simulink model "Control_Schematic_12"  (Simulink 8.3)
settings: Solver=ode4  StartTime=0.0  StopTime=35  FixedStep=Ts  RelTol=1e-3
values from neighbouring files (symbols this model uses):
  Aob1 = Am1 - Lob1'*Cm1    [StartUp_12.m]    (also in StartUp_12a.m)
  Aob2 = Am2 - Lob2'*Cm2    [StartUp_12.m]    (also in StartUp_12a.m)
  b = 156    [StartUp_10_Validation.m]    (also in StartUp_12.m; StartUp_12a.m; StartUp_2.m; StartUp_5.m)
  Bob1 = [Bm1 Lob1']    [StartUp_12.m]    (also in StartUp_12a.m)
  Bob2 = [Bm2 Lob2']    [StartUp_12.m]    (also in StartUp_12a.m)
  Cob1 = [1 0 0;0 1 0]    [StartUp_12.m]    (also in StartUp_12a.m)
  Cob2 = [1 0 0;0 1 0]    [StartUp_12.m]    (also in StartUp_12a.m)
  Dob1 = zeros(2,2)    [StartUp_12.m]    (also in StartUp_12a.m)
  Dob2 = zeros(2,2)    [StartUp_12.m]    (also in StartUp_12a.m)
  r = 50    [StartUp_10_Validation.m]    (also in StartUp_12.m; StartUp_12a.m; StartUp_2.m = 820; StartUp_5.m = 0.01)
  Ts = 1/100    (= 0.01)    [StartUp_10_Validation.m]    (also in StartUp_12.m; StartUp_12a.m; StartUp_2.m = 0.001; StartUp_5.m = 0.001)
undefined symbols (not defined in the file or in its folder): Beta_Correction
undefined symbols (not defined in the file): ADAMS_cwd, ADAMS_exec, ADAMS_host, ADAMS_init, ADAMS_inputs, ADAMS_outputs, ADAMS_prefix, ADAMS_static, ADAMS_sysdir
libraries: cstblocks x2, simulink x2
settings Model: Creator=baqumau  LastModifiedBy=baqumau
settings DataIOCC: SignalLoggingSaveFormat=Dataset
settings DebuggingCC: UnderspecifiedInitializationDetection=Simplified  StateNameClashWarn=none
settings GRTTargetCC: CombineOutputUpdateFcns=on  GRTInterface=off

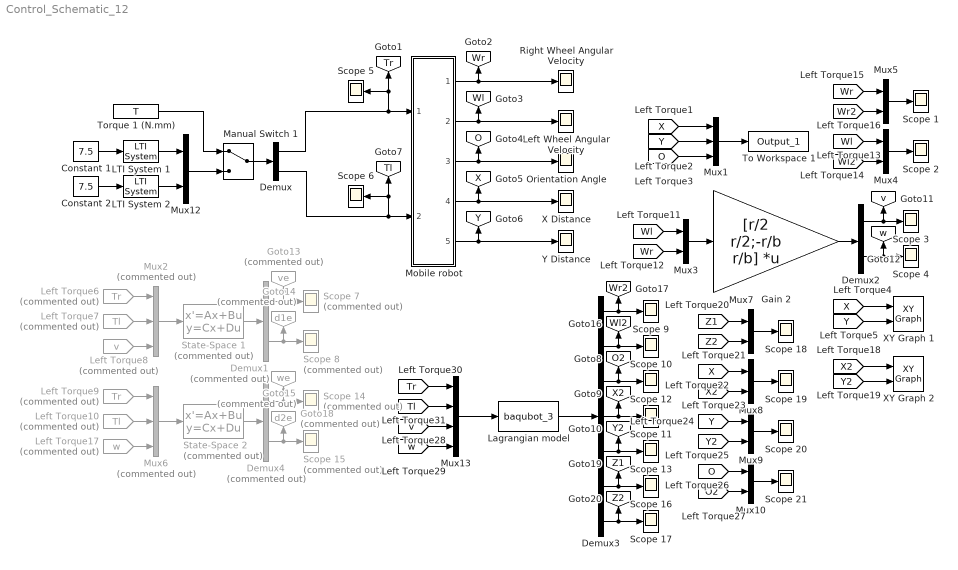
== system Control_Schematic_12 ==
  Constant 1 : Constant  Value=7.5
  Constant 2 : Constant  Value=7.5
  Demux : Demux  Outputs=2
  Demux1 : Demux  Commented=on  Outputs=2
  Demux2 : Demux  Outputs=2
  Demux3 : Demux  Outputs=7
  Demux4 : Demux  Commented=on  Outputs=2
  Gain 2 : Gain  Gain=[r/2 r/2;-r/b r/b]  Multiplication=Matrix(K*u)
  Goto13 : Goto  Commented=on  GotoTag=ve  TagVisibility=global
  Goto14 : Goto  Commented=on  GotoTag=d1e  TagVisibility=global
  Goto15 : Goto  Commented=on  GotoTag=we  TagVisibility=global
  Goto18 : Goto  Commented=on  GotoTag=d2e  TagVisibility=global
  LTI System 1 : cstblocks/LTI System  sys=Fz  IC=[]
  LTI System 2 : cstblocks/LTI System  sys=Fz  IC=[]
  Lagrangian model : S-Function  FunctionName=baqubot_3  Parameters=par  EnableBusSupport=off
  Left Torque10 : From  Commented=on  GotoTag=Tl  TagVisibility=global
  Left Torque17 : From  Commented=on  GotoTag=w  TagVisibility=global
  Left Torque6 : From  Commented=on  GotoTag=Tr  TagVisibility=global
  Left Torque7 : From  Commented=on  GotoTag=Tl  TagVisibility=global
  Left Torque8 : From  Commented=on  GotoTag=v  TagVisibility=global
  Left Torque9 : From  Commented=on  GotoTag=Tr  TagVisibility=global
  Left Wheel Angular Velocity : Scope
      settings: YMin=-1  YMax=1  SaveName=ScopeData2
  Manual Switch 1 : ManualSwitch
  Mobile robot : Subsystem
  Mux1 : Mux  Inputs=3
  Mux{3..5,7..10,12} (8 alike) : Mux  Inputs=2
  Mux13 : Mux
  Mux2 : Mux  Commented=on  Inputs=3
  Mux6 : Mux  Commented=on  Inputs=3
  Orientation Angle : Scope
      settings: YMin=-3  YMax=3
  Right Wheel Angular Velocity : Scope
      settings: YMin=-1  YMax=20  SaveName=ScopeData3
  Scope {1..6,9..13,16..21} (17 alike) : Scope
      Scope 1 settings: YMin=-10  YMax=20  SaveName=ScopeData15
      Scope 10 settings: YMin=0  YMax=5000  SaveName=ScopeData5
      Scope 11 settings: YMin=0  YMax=5000  SaveName=ScopeData9
      Scope 12 settings: YMin=0  YMax=5000  SaveName=ScopeData12
      Scope 13 settings: YMin=0  YMax=5000  SaveName=ScopeData13
      Scope 16 settings: YMin=0  YMax=5000  SaveName=ScopeData20
      Scope 17 settings: YMin=0  YMax=5000  SaveName=ScopeData21
      Scope 18 settings: YMin=-0.1  YMax=0.1  SaveName=ScopeData22
      Scope 19 settings: YMin=0  YMax=5000  SaveName=ScopeData23
      Scope 2 settings: YMax=50  SaveName=ScopeData14
      Scope 20 settings: YMin=0  YMax=5000  SaveName=ScopeData24
      Scope 21 settings: YMin=-15  YMax=2  SaveName=ScopeData25
      Scope 3 settings: YMin=0  YMax=5000  SaveName=ScopeData10
      Scope 4 settings: YMin=0  YMax=5000  SaveName=ScopeData11
      Scope 5 settings: YMin=0  YMax=5000  SaveName=ScopeData7
      Scope 6 settings: YMin=0  YMax=5000  SaveName=ScopeData8
      Scope 9 settings: YMin=-1  YMax=20  SaveName=ScopeData6
  Scope {7..8,14..15} (4 alike) : Scope  Commented=on
      Scope 14 settings: YMin=0  YMax=5000  SaveName=ScopeData18
      Scope 15 settings: YMin=0  YMax=5000  SaveName=ScopeData19
      Scope 7 settings: YMin=0  YMax=5000  SaveName=ScopeData16
      Scope 8 settings: YMin=0  YMax=5000  SaveName=ScopeData17
  State-Space 1 : StateSpace  Commented=on  A=Aob1  B=Bob1  C=Cob1  D=Dob1  X0=0
  State-Space 2 : StateSpace  Commented=on  A=Aob2  B=Bob2  C=Cob2  D=Dob2  X0=0
  To Workspace 1 : ToWorkspace  VariableName=Output_1  SaveFormat=Structure With Time  SampleTime=-1
  Torque 1 (N.mm) : FromWorkspace  VariableName=T  SampleTime=Ts  Interpolate=off  OutputAfterFinalValue=Holding final value
  X Distance : Scope
      settings: YMin=0  YMax=5000  SaveName=ScopeData4
  XY Graph 1 : simulink/Sinks/XY Graph  xmin=0  xmax=5000  ymin=0  ymax=5000  st=-1
  XY Graph 2 : simulink/Sinks/XY Graph  xmin=0  xmax=5000  ymin=0  ymax=5000  st=-1
  Y Distance : Scope
      settings: YMin=0  YMax=5000
  tag scope: O2=global, O=global, Tl=global, Tr=global, Wl2=global, Wl=global, Wr2=global, Wr=global, X2=global, X=global, Y2=global, Y=global, Z1=global, Z2=global, v=global, w=global
  wires:
  Mobile robot/1(Wrw) -> Right Wheel Angular Velocity/1, [Wr]
  Mobile robot/2(Wlw) -> Left Wheel Angular Velocity/1, [Wl]
  Mobile robot/3(Alpha) -> Orientation Angle/1, [O]
  Mobile robot/4(X_Dist) -> X Distance/1, [X]
  Mobile robot/5(Y_Dist) -> Y Distance/1, [Y]
  [X] -> Mux1/1
  [Y] -> Mux1/2
  [O] -> Mux1/3
  Mux1/1 -> To Workspace 1/1
  Demux/1 -> Mobile robot/1(Trw), Scope 5/1, [Tr]
  Demux/2 -> Mobile robot/2(Tlw), Scope 6/1, [Tl]
  [X] -> XY Graph 1/1
  [Y] -> XY Graph 1/2
  [Wl] -> Mux3/1
  [Wr] -> Mux3/2
  Mux3/1 -> Gain 2/1
  Gain 2/1 -> Demux2/1
  Demux2/2 -> Scope 4/1, [w]
  Demux2/1 -> Scope 3/1, [v]
  Mux4/1 -> Scope 2/1
  Mux5/1 -> Scope 1/1
  Manual Switch 1/1 -> Demux/1
  Torque 1 (N.mm)/1 -> Manual Switch 1/1
  Constant 1/1 -> LTI System 1/1
  Constant 2/1 -> LTI System 2/1
  LTI System 2/1 -> Mux12/2
  LTI System 1/1 -> Mux12/1
  Mux12/1 -> Manual Switch 1/2
  [Tr] -> Mux13/1
  Mux13/1 -> Lagrangian model/1
  [Tl] -> Mux13/2
  [v] -> Mux13/3
  [w] -> Mux13/4
  Demux3/1 -> Scope 9/1, [Wr2]
  Lagrangian model/1 -> Demux3/1
  [Wr] -> Mux5/1
  [Wl] -> Mux4/1
  Demux3/2 -> Scope 10/1, [Wl2]
  Demux3/3 -> Scope 12/1, [O2]
  Demux3/4 -> Scope 11/1, [X2]
  Demux3/5 -> Scope 13/1, [Y2]
  Mux2/1 -> State-Space 1/1
  Left Torque6/1 -> Mux2/1
  Left Torque7/1 -> Mux2/2
  Left Torque8/1 -> Mux2/3
  State-Space 1/1 -> Demux1/1
  Demux1/1 -> Scope 7/1, Goto13/1
  Demux1/2 -> Scope 8/1, Goto14/1
  Mux6/1 -> State-Space 2/1
  Left Torque9/1 -> Mux6/1
  Left Torque10/1 -> Mux6/2
  Left Torque17/1 -> Mux6/3
  State-Space 2/1 -> Demux4/1
  Demux4/1 -> Goto15/1, Scope 14/1
  Demux4/2 -> Goto18/1, Scope 15/1
  [Wr2] -> Mux5/2
  [Wl2] -> Mux4/2
  [X2] -> XY Graph 2/1
  [Y2] -> XY Graph 2/2
  Demux3/6 -> [Z1], Scope 16/1
  Demux3/7 -> Scope 17/1, [Z2]
  Mux7/1 -> Scope 18/1
  [Z1] -> Mux7/1
  [Z2] -> Mux7/2
  Mux8/1 -> Scope 19/1
  [X] -> Mux8/1
  [X2] -> Mux8/2
  Mux9/1 -> Scope 20/1
  [Y] -> Mux9/1
  [Y2] -> Mux9/2
  Mux10/1 -> Scope 21/1
  [O] -> Mux10/1
  [O2] -> Mux10/2

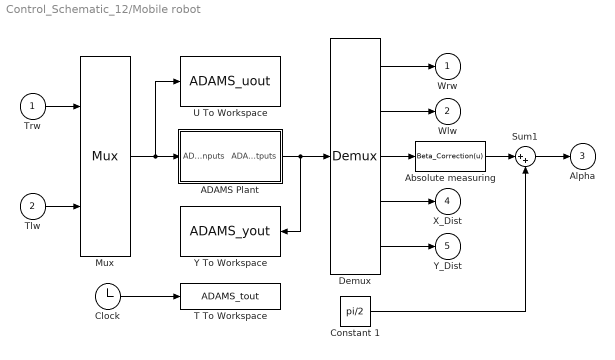
== system Control_Schematic_12/Mobile robot ==
  Trw : Inport
  Tlw : Inport  Port=2
  ADAMS Plant : Subsystem  LoadFcn=|  InitFcn=clear mex  mask(Adams Plant){exevie=ADAMS_sysdir, nam_in=ADAMS_inputs, namout=ADAMS_outputs, nampre=ADAMS_prefix, outfil=ADAMS_prefix, exesol=ADAMS_exec, stat=ADAMS_static, inicmd=[ADAMS_init], exetyp=C++, comtyp=PIPE(DDE), workdir=ADAMS_cwd, ada_host=ADAMS_host, modani=batch, modsim=discrete, dft=no, simulink_lead_cosim=yes, pin_interp_order=0, pout_extrap_order=0, pin_extrap_order=0, pout_interp_order=0, dt_out=Ts, o_rate=1, more=off}
      | %check based on dialog box setting for when setting by popup menu                                             
      | if exist('ADAMS_solver_type')                                                                                 
      |   if strcmp(ADAMS_solver_type,'C++')                                                                          
      |     set_param(gcb,'exetyp','C++');                                                                            
      |   else                                                                                                        
      |     set_param(gcb,'exetyp','Fortran');                                                                        
      |   end                                                                                                         
      | else                                                                                                          
      |   set_param(gcb,'exetyp','C++');                                                                              
      | end                                                                                                           
      | %set the mode if using acar_solver                                                                            
      | %REQUIRED HERE BECAUSE BELOW CAUSES MDLTERMINATE TO BE CALLED 2 TIMES IN MIDDLE OF SIMULATION WHEN SET IN MASK
      |                                                                                                               
      | %enable the direct feedthrough, sim mode, anim mode parameters by default                                     
      |                                                                                                               
      | if exist('set_some_params_states')                                                                            
      |                                                                                                               
      |   set_some_params_states({'dft','modsim','modani'},{'on','on','on'},'MaskEnables',gcb)                        
      |   %turn on direct feedthrough option                                                                          
      |   set_some_params_states({'dft'},{'on'},'MaskVisibilities',gcb)                                               
      |                                                                                                               
      |  end                                                                                                          
      |                                                                                                               
      |                                                                                                               
      | if exist('ADAMS_exec')                                                                                        
      |   if and(strcmp(get_param(gcb,'exesol'),'ADAMS_exec'),strcmp(ADAMS_exec,'acar_solver'))                       
      |     %set the sim mode to discrete -- only supported mode                                                      
      |     set_param(gcb,'modsim','discrete')                                                                        
      |      %turn off direct feedthrough option                                                                      
      |      set_some_params_states({'dft'},{'off'},'MaskVisibilities',gcb)                                           
      |     %set the animation mode to batch -- only supported mode                                                   
      |     set_param(gcb,'modani','batch')                                                                           
      |     %disable the direct feedthrough, sim mode, anim mode parameters                                           
      |     set_some_params_states({'modsim','modani'},{'off','off'},'MaskEnables',gcb)                               
      |   end                                                                                                         
      | end
      mask prompts: exevie "Adams install directory"; nam_in "Adams/View input names"; namout "Adams/View output names"; nampre "Adams model file prefix"; outfil "Output files prefix (opt.: if blank - no output)"; exesol "User executable (opt.: if blank - use standard)"; stat "Initial static simulation flag"; inicmd "Initialization commands"; exetyp "Adams/Solver type"; comtyp "Interprocess option"; workdir "Adams working directory"; ada_host "Adams host"; modani "Animation mode"; modsim "Simulation mode"; dft "Direct feedthrough"; simulink_lead_cosim "Discrete Computational Order - Simulink Leads Adams"; pin_interp_order "Plant input interpolation order"; pout_extrap_order "Plant output extrapolation order"; pin_extrap_order "Plant input extrapolation order"; pout_interp_order "Plant output interpolation order"; dt_out "Communication interval"; o_rate "Number of communications per output step"; more "More parameters"
      mask help: Simulate any Adams plant model either in Adams/Solver form (.adm file) or in Adams/View form (.cmd file)
      settings: OpenFcn=|
      | open_system(gcb,'mask')
      | if not(exist('set_some_params_states'))
      | 
      | warning('The script "set_some_params_states.m" cannot be found in the MATLAB PATH.  Cannot update the ADAMS Plant S-Function parameters.')
      | 
      | warning('Recommended action(optional):  run the Adams/Controls .m file first to help choose the correct settings in the Adams S-Function block.')
      | 
      | end
      mask Help:
      | <html>
      | This S-Function represents the non-linear Adams Plant with the inputs sent to the Adams model <br>
      |  and the outputs generated by the Adams model.  See the Adams/Controls documentation for more <br>
      | information.  This plant uses the following variables:<br>
      | <br>
      | <b>ADAMS_sysdir  :</b> Adams installation directory<br>
      | <b>ADAMS_inputs  :</b> Input variables View names vector<br>
      | <b>ADAMS_outputs :</b> Outputs variables View names vector<br>
      | <b>ADAMS_prefix  : </b>ADAMS model files prefix (.adm, .cmd); also doubles as output files prefix<br>
      | <b>ADAMS_exec :</b> Adams/Solver user library or keyword (e.g., acar_solver)<br>
      | <b>ADAMS_static :</b> yes|no - initial static before Co-simulation(discrete)/Function Evaluation(continuous)<br>
      | <b>ADAMS_init :</b>Initialization commands (i.e., Adams/View or Solver commands, depending on setting for Animation mode)<br>
      | <b>ADAMS_cwd : </b> Current working directory (for TCP/IP)<br>
      | <b>ADAMS_host : </b>Name of Adams server host (for TCP/IP)<br>
      | <b>ADAMS_mode :</b> Linear or non-linear (i.e., co-sim, function eval)<br>
      | <b>ADAMS_solver_type :</b>Fortran or C++ (used to set popup menu when first loaded) <br>
      | 
      | 
      | <br>
      | The following settings can be chosen:<br>
      | <br>
      | <b>Adams/Solver type:</b>  Fortran or C++ (will also set ADAMS_solver_type)<br>
      | <b>Interprocess option:</b> Pipe(DDE) or TCP/IP; TCP/IP can allow different machines run Adams and MATLAB<br>
      | <b>Animation mode:</b> batch (Solver, uses .adm) or interactive (View, uses .cmd)<br>
      | <b>Simulation mode:</b> discrete (Co-simulation) or continuous (Function Evaluation)<br>
      | <b>Discrete Computational Order - Simulink Lead Adams:</b> for discrete mode, chooses if Simulink leads the integration (yes) or lags (no);<br> if set to "no", can remove algebraic loop<br>
      | <b>Plant input interpolation order:</b> 0 = zero-order hold; 1 = linear (discrete mode only, where Simulink leads)<br>
      | <b>Plant output extrapolation order:</b> 0 = zero-order hold;1 = linear(discrete mode only, where Simulink leads)<br>
      | <b>Plant input extrapolation order:</b> 0 = zero-order hold; 1 = linear (discrete mode only, where Adams leads)<br>
      | <b>Plant output interpolation order:</b> 0 = zero-order hold;1 = linear(discrete mode only, where Adams leads)<br>
      | <b>Direct feedthrough:</b> yes|no - yes = Input directly effect output(continuous mode-only)<br>
      | <b>Communication interval:</b> Time step at which Co-simulation exchange information (e.g.,0.005); also controls <br>output for continuous mode (Function Evaluation)<br>
      | <b>Number of communications per output step: </b>Sets Adams output rate (.res, .req, .gra) integer value (default: 1)<br>
      | </html>
      mask Callback exesol:
      | if exist('set_some_params_states')
      | %enable the direct feedthrough, sim mode, anim mode parameters
      | set_some_params_states({'dft','modsim','modani'},{'on','on','on'},'MaskEnables',gcb)
      | %turn on direct feedthrough option
      | set_some_params_states({'dft'},{'on'},'MaskVisibilities',gcb)
      | end
      | 
      | if exist('ADAMS_exec')
      |   if and(strcmp(get_param(gcb,'exesol'),'ADAMS_exec'),strcmp(ADAMS_exec,'acar_solver'))
      |     %set the sim mode to discrete -- only supported mode
      |     %REMOVED:  BELOW CAUSES MDLTERMINATE TO BE CALLED 2 TIMES IN MIDDLE OF SIMULATION
      |     %Now in LoadFcn callback
      |     %set_param(gcb,'modsim','discrete')
      |      %turn off direct feedthrough option
      |     set_some_params_states({'dft'},{'off'},'MaskVisibilities',gcb)
      |     %set the animation mode to batch -- only supported mode
      |     %REMOVED:  BELOW CAUSES MDLTERMINATE TO BE CALLED 2 TIMES IN MIDDLE OF SIMULATION
      |     %Now in LoadFcn callback
      |     %set_param(gcb,'modani','batch')
      |     %disable the direct feedthrough, sim mode, anim mode parameters
      |     set_some_params_states({'modsim','modani'},{'off','off'},'MaskEnables',gcb)
      |   end
      | end
      mask TypeOptions exetyp: Fortran | C++
      mask Callback exetyp:
      | if strcmp(get_param(gcb,'exetyp'),'C++')
      |     ADAMS_solver_type='C++';
      | else
      |     ADAMS_solver_type='Fortran';
      | end
      mask TypeOptions comtyp: PIPE(DDE) | TCP/IP
      mask Callback comtyp:
      | if exist('set_some_params_states')
      | if strcmp(get_param(gcb,'comtyp'),'PIPE(DDE)')
      |     %turn off cwd, host options
      |     set_some_params_states({'ada_host','workdir'},{'off','off'},'MaskVisibilities',gcb)
      | else%if strcmp(get_param(gcb,'modsim'),'TCP/IP')
      |     %turn on cwd, host options
      |     set_some_params_states({'ada_host','workdir'},{'on','on'},'MaskVisibilities',gcb)
      | end
      | end
      mask TypeOptions modani: batch | interactive
      mask TypeOptions modsim: discrete | continuous
      mask Callback modsim:
      | if exist('set_some_params_states')
      | if strcmp(get_param(gcb,'modsim'),'discrete')
      |      %turn off direct feedthrough option
      |     set_some_params_states({'dft'},{'off'},'MaskVisibilities',gcb)
      |     %turn on discrete co-sim type if want to see more
      |     if strcmp(get_param(gcb,'more'),'on')
      |         set_some_params_states({'simulink_lead_cosim'},{'on'},'MaskVisibilities',gcb)
      |     end
      |     if strcmp(get_param(gcb,'simulink_lead_cosim'),'yes')
      |         %turn on interpolation/extrapolation options
      |         set_some_params_states({'pin_interp_order','pout_extrap_order',},{'on','on'},'MaskVisibilities',gcb)
      |     else
      |         set_some_params_states({'pin_extrap_order','pout_interp_order'},{'on','on'},'MaskVisibilities',gcb)
      |     end
      | else%if strcmp(get_param(gcb,'modsim'),'continuous')
      |      %turn off direct feedthrough option
      |     set_some_params_states({'dft'},{'on'},'MaskVisibilities',gcb)
      |     %turn off interpolation/extrapolation options
      |     set_some_params_states({'pin_interp_order','pout_extrap_order','pin_extrap_order','pout_interp_order','simulink_lead_cosim'},{'off','off','off','off','off'},'MaskVisibilities',gcb)
      | end
      | end
      mask TypeOptions dft: no | yes
      mask TypeOptions simulink_lead_cosim: yes | no
      mask Callback simulink_lead_cosim:
      | if exist('set_some_params_states')
      | if (strcmp(get_param(gcb,'simulink_lead_cosim'),'yes') && strcmp(get_param(gcb,'modsim'),'discrete'))
      |      %turn off unused interpolate/extrapolate options
      |     set_some_params_states({'pin_extrap_order','pout_interp_order'},{'off','off'},'MaskVisibilities',gcb)
      |     %turn on used interpolate/extrapolate options
      |     set_some_params_states({'pin_interp_order','pout_extrap_order'},{'on','on'},'MaskVisibilities',gcb)
      | elseif (strcmp(get_param(gcb,'simulink_lead_cosim'),'no') && strcmp(get_param(gcb,'modsim'),'discrete'))
      |     %turn on used interpolate/extrapolate options
      |     set_some_params_states({'pin_extrap_order','pout_interp_order'},{'on','on'},'MaskVisibilities',gcb)
      |      %turn off unused interpolate/extrapolate options
      |     set_some_params_states({'pin_interp_order','pout_extrap_order'},{'off','off'},'MaskVisibilities',gcb)
      | end
      | end
      mask TypeOptions pin_interp_order: 0 | 1
      mask TypeOptions pout_extrap_order: 0 | 1
      mask TypeOptions pin_extrap_order: 0 | 1
      mask TypeOptions pout_interp_order: 0 | 1
      mask Callback more:
      | if exist('set_some_params_states')
      | if (strcmp(get_param(gcb,'more'),'on'))
      |      %turn on infrequently used options
      |     set_some_params_states({'exevie','nam_in','namout','exesol','stat','inicmd'},{'on','on','on','on','on','on'},'MaskVisibilities',gcb)
      |     if strcmp(get_param(gcb,'modsim'),'discrete')
      |         set_some_params_states({'simulink_lead_cosim'},{'on'},'MaskVisibilities',gcb)
      |     end
      | elseif (strcmp(get_param(gcb,'more'),'off'))
      |     %turn off infrequently used options
      |     set_some_params_states({'exevie','nam_in','namout','exesol','stat','inicmd'},{'off','off','off','off','off','off'},'MaskVisibilities',gcb)
      |     if strcmp(get_param(gcb,'modsim'),'discrete')
      |         set_some_params_states({'simulink_lead_cosim'},{'off'},'MaskVisibilities',gcb)
      |     end
      | end
      | end
      mask Display: disp( 'MSC Software' )
  Absolute measuring : MATLABFcn  MATLABFcn=Beta_Correction(u)
  Clock : Clock
  Constant 1 : Constant  Value=pi/2
  Demux : Demux  Outputs=5
  Mux : Mux  Inputs=2
  Sum1 : Sum  Inputs=|++
  T To Workspace : ToWorkspace  VariableName=ADAMS_tout
      settings: MaxDataPoints=100000
  U To Workspace : ToWorkspace  VariableName=ADAMS_uout
      settings: MaxDataPoints=100000
  Y To Workspace : ToWorkspace  VariableName=ADAMS_yout
      settings: MaxDataPoints=100000
  Wrw : Outport
  Wlw : Outport  Port=2
  Alpha : Outport  Port=3
  X_Dist : Outport  Port=4
  Y_Dist : Outport  Port=5
  wires:
  Tlw/1 -> Mux/2
  Trw/1 -> Mux/1
  Demux/5 -> Y_Dist/1
  Demux/4 -> X_Dist/1
  Demux/2 -> Wlw/1
  Demux/1 -> Wrw/1
  ADAMS Plant/1(ADAMS outputs) -> Y To Workspace/1, Demux/1
  Mux/1 -> U To Workspace/1, ADAMS Plant/1(ADAMS inputs)
  Clock/1 -> T To Workspace/1
  Demux/3 -> Absolute measuring/1
  Absolute measuring/1 -> Sum1/1
  Sum1/1 -> Alpha/1
  Constant 1/1 -> Sum1/2

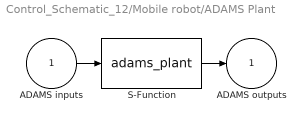
== system Control_Schematic_12/Mobile robot/ADAMS Plant ==
  ADAMS inputs : Inport
  S-Function : S-Function  StopFcn=clear mex  FunctionName=adams_plant  Parameters=exevie,exesol,stat,outfil,nampre,o_rate,nam_in,namout,dft,modsim,modani,dt_out,inicmd,exetyp,comtyp,ada_host, workdir,pin_interp_order,pout_extrap_order,pin_extrap_order,pout_interp_order,simulink_lead_cosim  EnableBusSupport=off
  ADAMS outputs : Outport  InitialOutput=0
  wires:
  S-Function/1 -> ADAMS outputs/1
  ADAMS inputs/1 -> S-Function/1
